simulink model "PandO"  (R2017a)
settings: Solver=VariableStepDiscrete  StartTime=0.0  StopTime=.02  RelTol=1e-3  EnableMultiTasking=on
libraries: powerlib x12, powerlib_extras x1, re_lib x1, simulink x1
settings Model: Creator=user  LastModifiedBy=acer
settings DataIOCC: LimitDataPoints=on  SaveFormat=Array
settings OptimizationCC: LifeSpan=inf
settings DebuggingCC: SFUnexpectedBacktrackingDiag=warning  SFNoUnconditionalDefaultTransitionDiag=warning  SFExecutionAtInitializationDiag=none
settings HardwareCC: ProdBitPerPointer=32  ProdBitPerSizeT=32  ProdBitPerPtrDiffT=32  ProdLargestAtomicFloat=None  ProdIntDivRoundTo=Undefined  ProdEndianess=Unspecified  ProdWordSize=32  ProdHWDeviceType=32-bit Generic
settings ModelReferenceCC: PropagateSignalLabelsOutOfModel=off
settings GRTTargetCC: TargetLangStandard=C89/C90 (ANSI)  GeneratePreprocessorConditionals=Disable all
settings ConfigComp: CovMetricSettings=dw  CovHtmlReporting=on  CovSaveCumulativeToWorkspaceVar=on  CovSaveSingleToWorkspaceVar=on  CovExternalEMLEnable=off

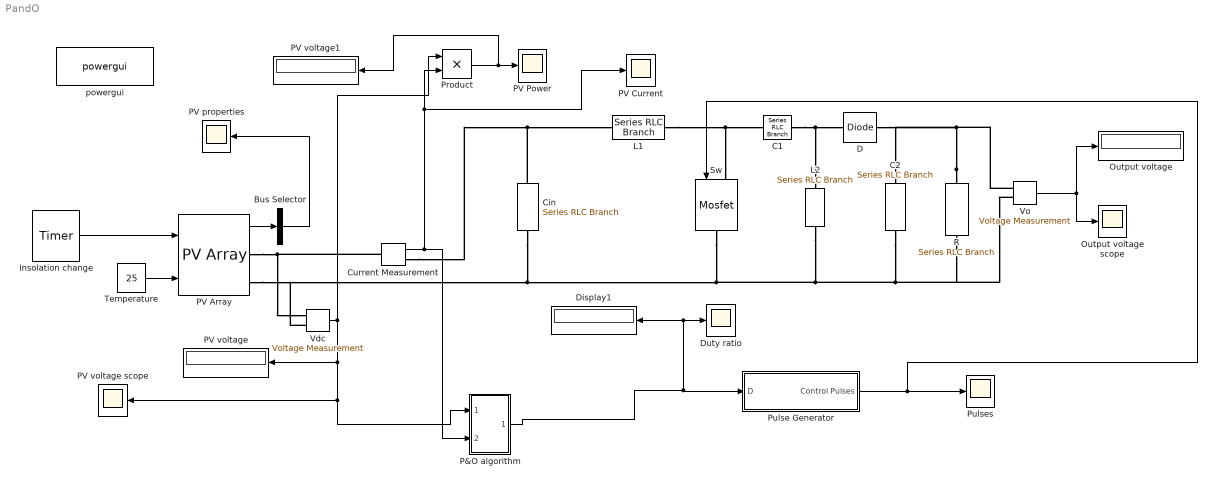
== system PandO ==
  Bus Selector : BusSelector  OutputSignals=V_PV,I_PV  OutputAsBus=on
  C1 : powerlib/Elements/Series RLC Branch  LConnTagsString=__new0  RConnTagsString=__new0  BranchType=C  Resistance=100  Inductance=1e-3  SetiL0=off  InitialCurrent=0  Capacitance=1e-6  Setx0=off  InitialVoltage=0  Measurements=None
  C2 : powerlib/Elements/Series RLC Branch  LConnTagsString=__new0  RConnTagsString=__new0  BranchType=C  Resistance=1  Inductance=1e-3  SetiL0=off  InitialCurrent=0  Capacitance=1.74e-6  Setx0=off  InitialVoltage=0  Measurements=None
  Cin : powerlib/Elements/Series RLC Branch  LConnTagsString=__new0  RConnTagsString=__new0  BranchType=C  Resistance=1  Inductance=1e-3  SetiL0=off  InitialCurrent=0  Capacitance=4.7e-6  Setx0=off  InitialVoltage=0  Measurements=None
  Current Measurement : powerlib/Measurements/Current Measurement  PhasorSimulation=off  OutputType=Complex  PSBequivalent=0
  D : powerlib/Power Electronics/Diode  Ron=0.001  Lon=0  Vf=.05  IC=0  UseSnubber=off  Rs=500  Cs=250e-9  Measurements=off
  Display1 : Display
  Duty ratio : Scope
  Insolation change : powerlib_extras/Control  Blocks/Timer  t="[0  .01]"  e="[270   480]"
  L1 : powerlib/Elements/Series RLC Branch  LConnTagsString=__new0  RConnTagsString=__new0  BranchType=L  Resistance=1  Inductance=22e-6  SetiL0=off  InitialCurrent=0  Capacitance=1e-6  Setx0=off  InitialVoltage=0  Measurements=None
  L2 : powerlib/Elements/Series RLC Branch  LConnTagsString=__new0  RConnTagsString=__new0  BranchType=L  Resistance=1  Inductance=22e-6  SetiL0=off  InitialCurrent=0  Capacitance=1e-6  Setx0=off  InitialVoltage=0  Measurements=None
  Output voltage : Display
  Output voltage scope : Scope
  P&O algorithm : Subsystem
  PV Array : re_lib/Solar/PV Array  Npar=9  Nser=2  PlotType=one module @ 25 deg.C & specified irradiances  S_vec=[270 480]  Temp_C_vec="[ 45 25  ]"  ModuleName=User-defined  PlotWhenSelected=off  Pm=16.2  Ncell=18  Voc=15  Isc=1.5  Vm=12  Im=1.35  beta_Voc_pc=-0.2941  alpha_Isc_pc=0.0681  beta_Voc=-0.044115  alpha_Isc=0.0010215  IL=1.5093  I0=4.0719e-12  nI=1.2209  Rsh=143.8293  Rs=0.95078  BAL=on  Tc=1e-6  Tfilter=2e-5
  PV Current : Scope
  PV Power : Scope
  PV properties : Scope
  PV voltage : Display
  PV voltage scope : Scope
  PV voltage1 : Display
  Product : Product
  Pulse Generator : Subsystem  mask{F=50e3}
      mask prompts: F "Carrier Frequency"
  Pulses : Scope
  R : powerlib/Elements/Series RLC Branch  LConnTagsString=__new0  RConnTagsString=__new0  BranchType=R  Resistance=10  Inductance=1e-3  SetiL0=off  InitialCurrent=0  Capacitance=1e-6  Setx0=off  InitialVoltage=0  Measurements=None
  Sw : powerlib/Power Electronics/Mosfet  Ron=0.1  Lon=0  Rd=0.01  Vfd=0  IC=0  Rs=1e5  Cs=inf  Measurements=off
  Temperature : Constant  Value=25  VectorParams1D=off  SampleTime=2e-5
  "Vdc " : powerlib/Measurements/Voltage Measurement  Tag=PoWeRsYsTeMmEaSuReMeNt  PhasorSimulation=off  OutputType=Magnitude  PSBequivalent=0
  Vo : powerlib/Measurements/Voltage Measurement  PhasorSimulation=off  OutputType=Complex  PSBequivalent=0
  powergui : powerlib/powergui  Priority=1  SimulationMode=Discrete  SampleTime=50e-6  frequency=50  Iterations=50  frequencyindice=0  Pbase=100e6  ErrMax=1e-4  UnitsV=kV  UnitsW=MW  buscounter=0  FunctionMessages=off  echomessages=off  EnableUseOfTLC=off  CurrentSourceSwitches=off  DisableSnubberDevices=off  DisableRonSwitches=off  DisableVfSwitches=on  DisplayEquations=off  SolverType=Tustin/Backward Euler (TBE)  Interpol=off  ExternalGateDelay=off  methode=off  Ts=0  x0status=blocks  SPID=on  SwTol=0  HookPort=off  RestoreLinks=warning  ResistiveCurrentMeasurement=off  Frange=[0:2:500]  Ylog=off  Xlog=on  ShowGrid=off  save=off  variable=ZData  structure=0  ZoomFFT=on  StartTime=0.0  cycles=1  DisplayStyle=1  fundamental=60  FreqAxis=off  MaxFrequency=1000  frequencyindicesteady=1  RmsSteady=1  display=off
  wires:
  PV Array/1 -> Bus Selector/1
  Vo/1 -> Output voltage scope/1, Output voltage/1
  P&O algorithm/1(duty) -> Duty ratio/1, Display1/1, Pulse Generator/1(D)
  Pulse Generator/1(Control Pulses) -> Sw/1, Pulses/1
  Bus Selector/1 -> PV properties/1
  Temperature/1 -> PV Array/2
  "Vdc "/1 -> PV voltage/1, P&O algorithm/1(Vpv), PV voltage scope/1, Product/1
  Current Measurement/1 -> P&O algorithm/2(Ipv), PV Current/1, Product/2
  Insolation change/1 -> PV Array/1
  Product/1 -> PV voltage1/1, PV Power/1
  connections:
  Sw/RConn1 -- Cin/RConn1 -- PV Array/RConn2 -- "Vdc "/LConn2 -- L2/RConn1 -- C2/RConn1 -- Vo/LConn2 -- R/RConn1
  L1/RConn1 -- C1/LConn1 -- Sw/LConn1
  R/LConn1 -- Vo/LConn1 -- C2/LConn1 -- D/RConn1
  C1/RConn1 -- D/LConn1 -- L2/LConn1
  Current Measurement/RConn1 -- Cin/LConn1 -- L1/LConn1
  Current Measurement/LConn1 -- PV Array/RConn1 -- "Vdc "/LConn1

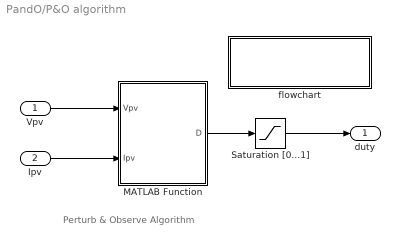
== system PandO/P&O algorithm ==
  note: Perturb & Observe Algorithm
  Vpv : Inport  OutDataTypeStr=double  PortDimensions=1  SampleTime=[0.0001,0]
  Ipv : Inport  Port=2  OutDataTypeStr=double  PortDimensions=1  SampleTime=[0.0001,0]
  MATLAB Function : MATLAB Function  TreatAsAtomicUnit=on
  Saturation [0...1] : Saturate  UpperLimit=1  LowerLimit=0  LinearizeAsGain=off
  flowchart : Subsystem
      settings: OpenFcn=winopen('PnO.jpg');
      mask Display: disp('Algorithm\nFlowchart')
  duty : Outport  OutDataTypeStr=double  PortDimensions=1  SampleTime=[0.0001,0]
  wires:
  Saturation [0...1]/1 -> duty/1
  MATLAB Function/1(D) -> Saturation [0...1]/1
  Ipv/1 -> MATLAB Function/2(Ipv)
  Vpv/1 -> MATLAB Function/1(Vpv)

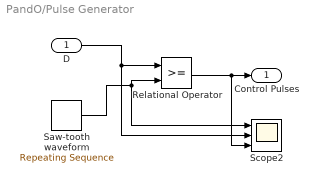
== system PandO/Pulse Generator ==
  D : Inport
  Relational Operator : RelationalOperator  OutDataTypeStr=boolean  RndMeth=Nearest
  Saw-tooth waveform : simulink/Sources/Repeating Sequence  rep_seq_t=[0 0.5 1]/F  rep_seq_y=[0 1 0]
  Scope2 : Scope  NumInputPorts=3
  Control Pulses : Outport
  wires:
  Saw-tooth waveform/1 -> Relational Operator/2, Scope2/1
  Relational Operator/1 -> Scope2/3, Control Pulses/1
  D/1 -> Relational Operator/1, Scope2/2

== system PandO/P&O algorithm/flowchart ==

== matlab function PandO/P&O algorithm/MATLAB Function ==
  settings: updateMethod=DISCRETE  sampleTime=1e-4
  data: Vpv input; D output; Ipv input
function D = PandO(Vpv,Ipv)

persistent Dprev Pprev Vprev

% Initialize the internal values for the voltage and power on the
% first pass
 if isempty(Dprev)
     Dprev = .58;
     Vprev = 12;
     Pprev = 16.2;
 end

% Initialize algorithm parameters
deltaD = 0.00025;

% Calculate measured array power
Ppv = Vpv*Ipv;

% Increase or decrease duty cycle based on conditions
if (Ppv-Pprev) ~= 0
    if (Ppv-Pprev) > 0
        if (Vpv-Vprev) > 0
            D = Dprev - deltaD;
        else
            D = Dprev + deltaD;
        end
    else
        if (Vpv-Vprev) > 0
            D = Dprev + deltaD;
        else
            D = Dprev - deltaD;
        end        
    end
else
    D = Dprev;
end


disp(D);
% Update internal values
Dprev = D;
Vprev = Vpv;
Pprev = Ppv;
